simulink model "Planta"  (R2024a)
settings: Solver=VariableStepAuto  StartTime=0.0  StopTime=3  RelTol=1e-3
undefined symbols (not defined in the file): DenZ, k, NumZ, p, Ts, z
settings Model: Creator=cesar  LastModifiedBy=cesar

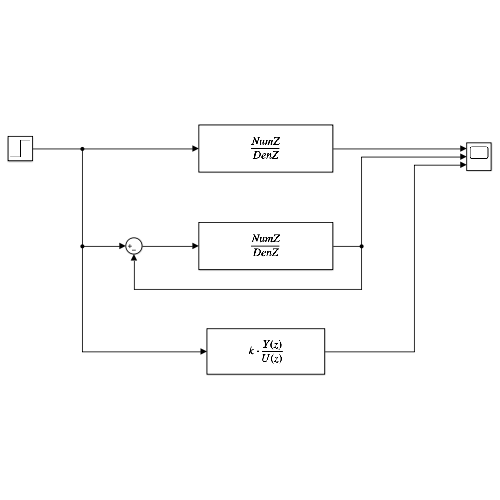
[thumbnail: Simulink's stored preview of the top-level diagram]
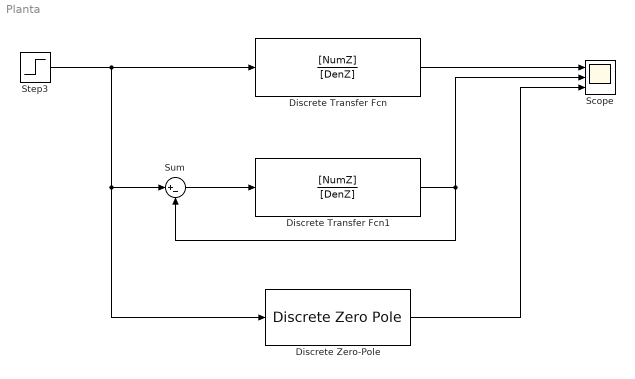
== system Planta ==
  Discrete Transfer Fcn : DiscreteTransferFcn  Numerator=[NumZ]  Denominator=[DenZ]  SampleTime=0.01
  Discrete Transfer Fcn1 : DiscreteTransferFcn  Numerator=[NumZ]  Denominator=[DenZ]  SampleTime=0.01
  Discrete Zero-Pole : DiscreteZeroPole  Zeros=z  Poles=p  Gain=k  SampleTime=Ts
  Scope : Scope  NumInputPorts=3
  Step3 : Step  Time=0  SampleTime=0
  Sum : Sum  Inputs=|+-
  wires:
  Step3/1 -> Discrete Zero-Pole/1, Sum/1, Discrete Transfer Fcn/1
  Discrete Transfer Fcn/1 -> Scope/1
  Discrete Transfer Fcn1/1 -> Sum/2, Scope/2
  Sum/1 -> Discrete Transfer Fcn1/1
  Discrete Zero-Pole/1 -> Scope/3
